simulink subsystem "Actuator_Models_2"  (R2026a)
settings: Solver=VariableStepAuto
undefined symbols (not defined in the file): DiscIntNeverNeededParam, distMode, dt_SIM, u0
settings Model: Creator=pplat  LastModifiedBy=pplat

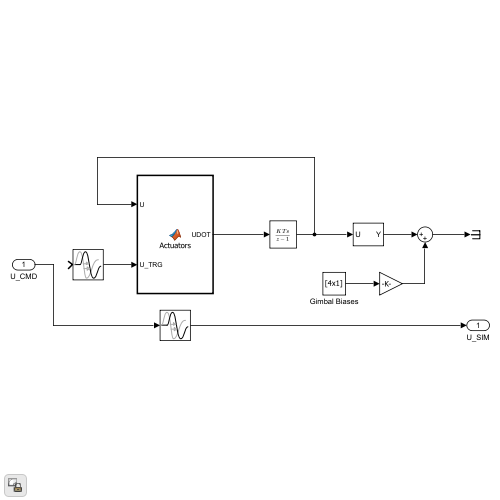
[thumbnail: Simulink's stored preview of the top-level diagram]
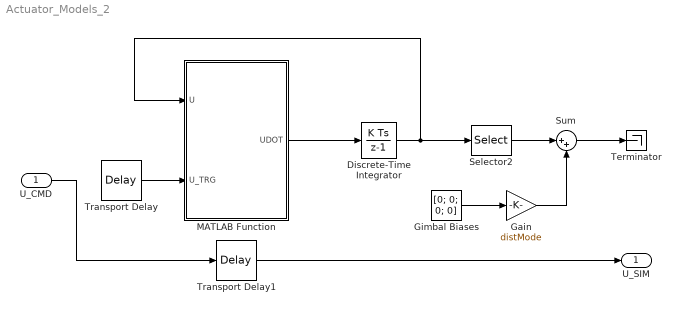
== system Actuator_Models_2 ==
  U_CMD : Inport  OutDataTypeStr=double  PortDimensions=[4,1]
  Discrete-Time Integrator : DiscreteIntegrator  InitialCondition=[zeros(4,1); u0(3); 0]  SampleTime=dt_SIM  ICPrevOutput=DiscIntNeverNeededParam  ICPrevScaledInput=DiscIntNeverNeededParam
  Gain : Gain  Gain=distMode
  Gimbal Biases : Constant  Value=[0; 0; 0; 0]  VectorParams1D=off
  MATLAB Function : MATLAB Function  TreatAsAtomicUnit=on
  Selector2 : Selector  IndexOptions=Index vector (dialog)  Indices=[1 3 5 6]  OutputSizes=1
  Sum : Sum  Inputs=|++
  Terminator : Terminator
  Transport Delay : TransportDelay  DelayTime=0.02  InitialOutput=u0
  Transport Delay1 : TransportDelay  DelayTime=0.02  InitialOutput=u0
  U_SIM : Outport  OutDataTypeStr=double  PortDimensions=[4,1]
  wires:
  Selector2/1 -> Sum/1
  Gain/1 -> Sum/2
  Sum/1 -> Terminator/1
  MATLAB Function/1(UDOT) -> Discrete-Time Integrator/1
  Gimbal Biases/1 -> Gain/1
  Discrete-Time Integrator/1 -> Selector2/1, MATLAB Function/1(U)
  Transport Delay/1 -> MATLAB Function/2(U_TRG)
  U_CMD/1 -> Transport Delay1/1
  Transport Delay1/1 -> U_SIM/1

== matlab function Actuator_Models_2/MATLAB Function ==
  data: U input size=[6, 1]; UDOT output size=[6, 1]; U_TRG input size=[4, 1]
function UDOT = Actuators(U, U_TRG)
    UDOT = zeros(6, 1);
    
    a = 800;
    b = 70;
    k1 = 0;
    k2 = 0;
    tau = 0.15;

    theta_error = k1 * (1 - cos(U(1)));
    phi_error = k2 * (1 - cos(U(3)));

    % Use local variables instead of modifying the read-only input 'U'
    u_mod_3 = U(3) - theta_error;
    u_mod_1 = U(1) - phi_error;

    % Explicitly assign each element to prevent Coder slicing errors
    UDOT(1) = U(2);
    UDOT(2) = a * (U_TRG(1) - u_mod_1) - b * U(2);
    UDOT(3) = U(4);
    UDOT(4) = a * (U_TRG(2) - u_mod_3) - b * U(4);
    UDOT(5) = (1/tau) * (U_TRG(3) - U(5));
    UDOT(6) = (1/(tau/2)) * (U_TRG(4) - U(6));
end
